simulink model "testat_2_a2"  (R2016a)
settings: Solver=VariableStepAuto  StartTime=0.0  StopTime=20  MaxStep=0.01  RelTol=1e-3
values from neighbouring files (symbols this model uses):
  c = 1.2    [testat2_a1.m]
  D = 1.2    [testat2_a1.m]
  m = 4.5    [testat2_a1.m]
  y0 = 1    [testat2_a1.m]
settings Model: Creator=bachman0  LastModifiedBy=bachman0

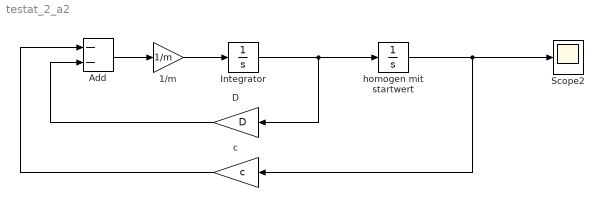
== system testat_2_a2 ==
  1/m : Gain  Gain=1/m
  Add : Sum  Inputs=--
  "D\t" : Gain  Gain=D
  Integrator : Integrator
  Scope2 : Scope
  c : Gain  Gain=c
  homogen mit startwert : Integrator  InitialCondition=y0
  wires:
  Integrator/1 -> "D\t"/1, homogen mit startwert/1
  homogen mit startwert/1 -> c/1, Scope2/1
  "D\t"/1 -> Add/2
  c/1 -> Add/1
  Add/1 -> 1/m/1
  1/m/1 -> Integrator/1
